simulink model "Flowchart2"  (Simulink 6.0)
settings: Solver=FixedStepDiscrete  StartTime=0.0  StopTime=10.0  RelTol=1e-3
settings Model: Creator=scaife  LastModifiedBy=scaife  ExtModeAutoUpdateStatusClock=off

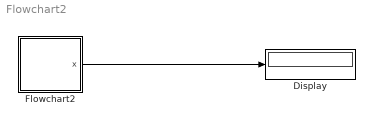
== system Flowchart2 ==
  Display : Display
  Flowchart2 : Stateflow chart
  wires:
  Flowchart2/1(x) -> Display/1

== stateflow chart Flowchart2 ==
  state A
    (default) -> (junction 4) : {x++;}
  data: x output int32
